simulink model "Exp_10"  (R2021a)
settings: Solver=VariableStepDiscrete  StartTime=0.0  StopTime=0.04  MaxStep=0.0008  RelTol=1e-3
libraries: spsDiodeLib x6, spsThreePhaseProgrammableVoltageSourceLib x1, spsThreePhaseVIMeasurementLib x1, spsGroundLib x1, spsVoltageMeasurementLib x1, spsSeriesRLCBranchLib x1, spsCurrentMeasurementLib x1, spspowerguiLib x1
settings Model: Creator=Mehedi  LastModifiedBy=DCL
settings SolverCC: AlgebraicLoopSolver=TrustRegion
settings DataIOCC: ReturnWorkspaceOutputs=off
settings DebuggingCC: SFMachineParentedDataDiag=warning  ArithmeticOperatorsInVariantConditions=warning
settings SFSimCC: SimUseLocalCustomCode=off  CustomCodeUndefinedFunction=UseInterfaceOnly
settings RTWCC: RTWUseLocalCustomCode=off

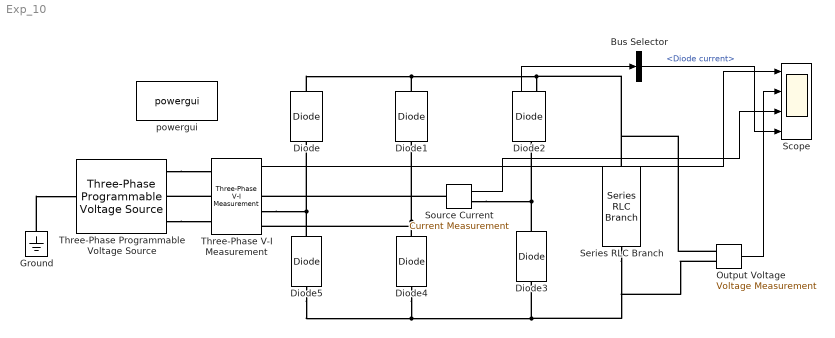
== system Exp_10 ==
  " Scope" : Scope  NumInputPorts=4
  " Three-Phase Programmable Voltage Source" : spsThreePhaseProgrammableVoltageSourceLib/Three-Phase Programmable Voltage Source  PositiveSequence="[220  0 50]"  VariationEntity=Amplitude  VariationType=Table of time-amplitude pairs  VariationTypeAlt=Step  VariationStep=0.5  VariationRate=10  VariationMagnitude=0.3  VariationFrequency=2  VariationTiming=[1 2]  VariationPhaseA=off  Amplitudes=[1 0.8 1.2 1.0]  TimeValues=[0 0.1 0.15 0.2]  HarmonicGeneration=off  HarmonicA=[3 0.2 -25 0]  HarmonicB=[2 0.15 35 2]  Timing="[0.05  3]"  BusType=swing  Pref=0  Qref=0  Qmin=-inf  Qmax=inf
  " Three-Phase V-I Measurement" : spsThreePhaseVIMeasurementLib/Three-Phase V-I Measurement  VoltageMeasurement=phase-to-ground  SetLabelV=off  LabelV=Vabc  Vpu=off  VpuLL=off  CurrentMeasurement=yes  SetLabelI=off  LabelI=Iabc  Ipu=off  Pbase=100e6  Vbase=500e3  OutputType=Complex  PhasorSimulation=off  PSBequivalent=0
   Diode{,1,3..5} (5 alike) : spsDiodeLib/Diode  Ron=0.001  Lon=0  Vf=0.8  IC=0  UseSnubber=0  Rs=500  Cs=250e-9  Measurements=off
  " Diode2" : spsDiodeLib/Diode  Ron=0.001  Lon=0  Vf=0.8  IC=0  UseSnubber=0  Rs=500  Cs=250e-9  Measurements=on
  Bus Selector : BusSelector  OutputSignals=Diode current
  Ground : spsGroundLib/Ground  LConnTagsString=a
  Output Voltage : spsVoltageMeasurementLib/Voltage Measurement  PhasorSimulation=off  OutputType=Complex  PSBequivalent=0
  Series RLC Branch : spsSeriesRLCBranchLib/Series RLC Branch  LConnTagsString=__new0  RConnTagsString=__new0  BranchType=R  Resistance=10  Inductance=1e-3  SetiL0=off  InitialCurrent=0  Capacitance=1e-6  Setx0=off  InitialVoltage=0  Measurements=None
  Source Current : spsCurrentMeasurementLib/Current Measurement  PhasorSimulation=off  OutputType=Complex  PSBequivalent=0
  powergui : spspowerguiLib/powergui  Priority=1  SimulationMode=Discrete  SampleTime=50e-6  frequency=50  Iterations=50  frequencyindice=50  Pbase=100e6  ErrMax=1e-4  UnitsV=kV  UnitsW=MW  buscounter=0  FunctionMessages=off  echomessages=off  EnableUseOfTLC=off  CurrentSourceSwitches=off  DisableSnubberDevices=off  DisableRonSwitches=off  DisableVfSwitches=off  DisplayEquations=off  AutomaticDiscreteSolvers=off  SolverType=Tustin/Backward Euler (TBE)  Interpol=off  ExternalGateDelay=off  methode=off  Ts=100  x0status=blocks  SPID=on  SwTol=0  HookPort=off  NonlinearTolerance=1e-4  nMaxIteration=100  ContinueOnMaxIteration=off  RestoreLinks=warning  ResistiveCurrentMeasurement=off  Frange=[0:2:500]  Ylog=off  Xlog=on  ShowGrid=off  save=off  variable=ZData  structure=0  ZoomFFT=off  StartTime=0.0  cycles=1  DisplayStyle=1  fundamental=60  FreqAxis=off  MaxFrequency=1000  frequencyindicesteady=1  RmsSteady=1  display=off
  wires:
  " Three-Phase V-I Measurement"/1 -> " Scope"/1
  Output Voltage/1 -> " Scope"/2
  Source Current/1 -> " Scope"/3
  " Diode2"/1 -> Bus Selector/1
  Bus Selector/1 -> " Scope"/4  "<Diode current>"
  connections:
  " Three-Phase V-I Measurement"/LConn2 -- " Three-Phase Programmable Voltage Source"/RConn2
  " Three-Phase Programmable Voltage Source"/RConn1 -- " Three-Phase V-I Measurement"/LConn1
  " Three-Phase Programmable Voltage Source"/RConn3 -- " Three-Phase V-I Measurement"/LConn3
  " Diode5"/RConn1 -- " Three-Phase V-I Measurement"/RConn2 -- " Diode"/LConn1
  " Diode3"/RConn1 -- Source Current/RConn1 -- " Diode2"/LConn1
  " Diode5"/LConn1 -- " Diode4"/LConn1 -- Series RLC Branch/RConn1 -- Output Voltage/LConn2 -- " Diode3"/LConn1
  " Diode"/RConn1 -- " Diode1"/RConn1 -- Output Voltage/LConn1 -- Series RLC Branch/LConn1 -- " Diode2"/RConn1
  Ground/LConn1 -- " Three-Phase Programmable Voltage Source"/LConn1
  " Diode4"/RConn1 -- " Three-Phase V-I Measurement"/RConn3 -- " Diode1"/LConn1
  Source Current/LConn1 -- " Three-Phase V-I Measurement"/RConn1
